simulink subsystem "Controller"  (R2025b)
settings: Solver=VariableStepAuto  StartTime=0.0  StopTime=10.0  RelTol=1e-3
values from neighbouring files (symbols this model uses):
  Feedforward = 0    [EReg_N2O_Simulink_Init.m]    (also in EReg_Tank_Drain_Init.m)
  K_D = 3    [EReg_N2O_Simulink_Init.m]    (also in EReg_Tank_Drain_Init.m = 8; EReg_Tank_Drain_N2O_Sim.m = params.K_D)
  K_I = 15    [EReg_N2O_Simulink_Init.m]    (also in EReg_Tank_Drain_Init.m = 2; EReg_Tank_Drain_N2O_Sim.m = params.K_I)
  K_P = 20    [EReg_N2O_Simulink_Init.m]    (also in EReg_Tank_Drain_Init.m = 8; EReg_Tank_Drain_N2O_Sim.m = params.K_P)
  N = 100    [EReg_N2O_Simulink_Init.m]    (also in EReg_Tank_Drain_Init.m)
libraries: simulink x2, slpidlib x1
settings Model: Creator=anzashoaib  LastModifiedBy=Rocklord

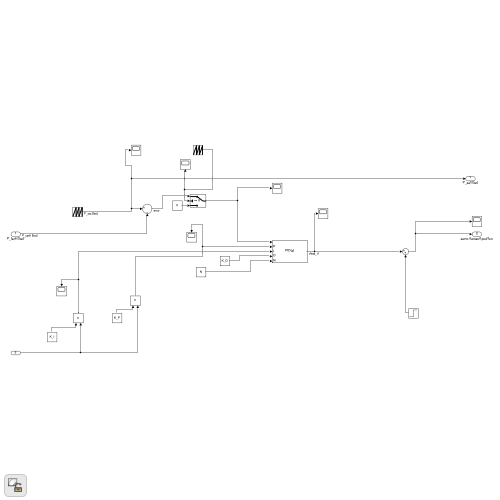
[thumbnail: Simulink's stored preview of the top-level diagram]
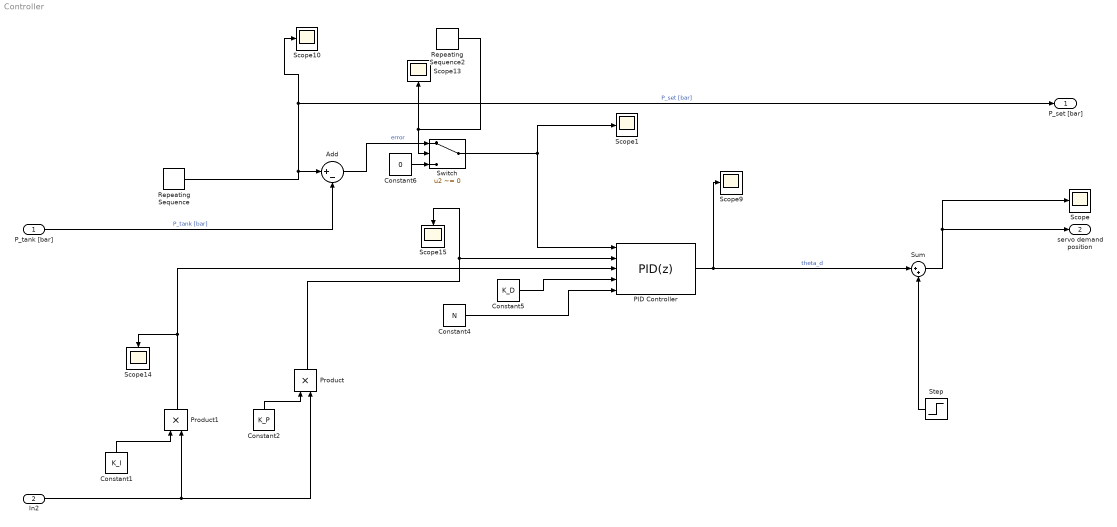
== system Controller ==
  P_tank [bar] : Inport  OutDataTypeStr=double  PortDimensions=1  SampleTime=0
  In2 : Inport  Port=2  OutDataTypeStr=double  PortDimensions=1  SampleTime=0
  Add : Sum  Inputs=|+-
  Constant1 : Constant  Value=K_I
  Constant2 : Constant  Value=K_P
  Constant4 : Constant  Value=N
  Constant5 : Constant  Value=K_D
  Constant6 : Constant  Value=0
  PID Controller : slpidlib/PID Controller  Controller=PID  Form=Parallel  TimeDomain=Discrete-time  UseExternalTs=off  SampleTime=-1  IntegratorMethod=Forward Euler  FilterMethod=Forward Euler  ControllerParametersSource=external  P=1.5  I=3  UseKiTs=off  D=0  UseExternalDerivativeSource=off  N=100  UseFilter=on  TunerSelectOption=Transfer Function Based (PID Tuner App)  InitialConditionSource=internal  InitialConditionForIntegrator=0  InitialConditionForFilter=0  DifferentiatorICPrevScaledInput=0  ExternalReset=none  TrackingMode=off  Kt=1  LimitOutput=off  SatLimitsSource=internal  UpperSaturationLimit=180  LowerSaturationLimit=0  LinearizeAsGain=on  AntiWindupMode=clamping  Kb=1  LimitIntegrator=on  UpperIntegratorSaturationLimit=20  LowerIntegratorSaturationLimit=-20  POutMin=[]  POutMax=[]  IOutMin=[]  IOutMax=[]  DOutMin=[]  DOutMax=[]  NOutMin=[]  NOutMax=[]  SumOutMin=[]  SumOutMax=[]  SaturationOutMin=[]  SaturationOutMax=[]  PParamMin=[]  PParamMax=[]  IParamMin=[]  IParamMax=[]  DParamMin=[]  DParamMax=[]  NParamMin=[]  NParamMax=[]  KbParamMin=[]  KbParamMax=[]  KtParamMin=[]  KtParamMax=[]  KbOutMin=[]  KbOutMax=[]  KtOutMin=[]  KtOutMax=[]  IntegratorOutMin=[]  IntegratorOutMax=[]  FilterOutMin=[]  FilterOutMax=[]  SumI1OutMin=[]  SumI1OutMax=[]  SumI2OutMin=[]  SumI2OutMax=[]  SumI3OutMin=[]  SumI3OutMax=[]  SumI4OutMin=[]  SumI4OutMax=[]  SumDOutMin=[]  SumDOutMax=[]  DifferentiatorOutMin=[]  DifferentiatorOutMax=[]  FilterDiffOutCoefMin=[]  FilterDiffOutCoefMax=[]  ReciprocalOutMin=[]  ReciprocalOutMax=[]  SumDenOutMin=[]  SumDenOutMax=[]  SumNumOutMin=[]  SumNumOutMax=[]  DivideOutMin=[]  DivideOutMax=[]  UdiffTsProdOutMin=[]  UdiffTsProdOutMax=[]  NTsProdOutMin=[]  NTsProdOutMax=[]  UintegralTsProdOutMin=[]  UintegralTsProdOutMax=[]  UngainTsProdOutMin=[]  UngainTsProdOutMax=[]  ClampingZeroOutDataTypeStr=Inherit: Inherit via back propagation  ClampingZeroOutMin=[]  ClampingZeroOutMax=[]  FilterDenConstantOutDataTypeStr=Inherit: Inherit via back propagation  FilterDenConstantOutMin=[]  FilterDenConstantOutMax=[]  PCopyOutDataTypeStr=Inherit: Inherit via back propagation  PCopyOutMin=[]  PCopyOutMax=[]  NCopyOutDataTypeStr=Inherit: Inherit via back propagation  NCopyOutMin=[]  NCopyOutMax=[]  IntegratorContinuousStateAttributes=''  IntegratorStateMustResolveToSignalObject=off  IntegratorRTWStateStorageClass=Auto  FilterContinuousStateAttributes=''  FilterStateMustResolveToSignalObject=off  FilterRTWStateStorageClass=Auto  ParallelPVariant=ExternalParameters  IdealPVariant=Disabled  IVariant=ExternalParameters  DVariant=ExternalParameters  IntegratorVariant=Discrete  SatVariant=Disabled  AWVariant=Passthrough  PCopyVariant=Disabled  TRVariant=Disabled  FdbkBlocksVariant=Forward  IdealPFdbkVariant=Disabled  SatFdbkVariant=Disabled  DerivativeFilterVariant=ForwardEulerFilter  NVariant=ExternalParameters  NCopyVariant=Disabled  FilterICVariant=InternalICsFilter  IntegratorICVariant=InternalICs  ExternalResetVariant=Disabled  TRSumVariant=Passthrough  SumFdbkVariant=Disabled  SumVariant=Sum_PID  TsampFilterVariant=InternalTs  TsampNgainVariant=Passthrough  TsampIntegralVariant=Disabled_SignalSpec  ExternalSaturationOutDataTypeStr=Inherit: Same as second input  DerivativeSourceVariant=ErrorSignal  PreIntVariant=InternalPreInt
  Product : Product
  Product1 : Product
  Repeating Sequence : simulink/Sources/Repeating Sequence  rep_seq_t=time  rep_seq_y=setpoint
  Repeating Sequence2 : simulink/Sources/Repeating Sequence  rep_seq_t=time  rep_seq_y=controller_on_setpoint
  Scope{,1,9..10,13..15} (7 alike) : Scope
      Scope settings: ActiveDisplayYMinimum=-1688.77171  ActiveDisplayYMaximum=357.47639  DataLoggingVariableName=ScopeData7
      Scope1 settings: ActiveDisplayYMinimum=-2.28363  ActiveDisplayYMaximum=0.62203  DataLoggingVariableName=ScopeData9
      Scope10 settings: ActiveDisplayYMinimum=51.3375  ActiveDisplayYMaximum=67.98472  DataLoggingVariableName=ScopeData10
      Scope13 settings: ActiveDisplayYMinimum=-0.125  ActiveDisplayYMaximum=1.125  DataLoggingVariableName=ScopeData11
      Scope14 settings: ActiveDisplayYMinimum=5.20102  ActiveDisplayYMaximum=13.19086  DataLoggingVariableName=ScopeData12
      Scope15 settings: ActiveDisplayYMinimum=13.00254  ActiveDisplayYMaximum=32.97714  DataLoggingVariableName=ScopeData13
      Scope9 settings: ActiveDisplayYMinimum=-1660.50954  ActiveDisplayYMaximum=362.9195  DataLoggingVariableName=ScopeData14
  Step : Step  After=Feedforward  SampleTime=0
  Sum : Sum  Inputs=|++
  Switch : Switch  Criteria=u2 ~= 0  SaturateOnIntegerOverflow=off  InputSameDT=off
  P_set [bar] : Outport  OutDataTypeStr=double  PortDimensions=1  SampleTime=0
  servo demand position : Outport  Port=2  OutDataTypeStr=double  PortDimensions=1  SampleTime=0
  wires:
  Product1/1 -> PID Controller/3, Scope14/1
  Product/1 -> PID Controller/2, Scope15/1
  Constant4/1 -> PID Controller/5
  Constant2/1 -> Product/1
  PID Controller/1 -> Sum/1, Scope9/1  "theta_d"
  P_tank [bar]/1 -> Add/2  "P_tank [bar]"
  Constant6/1 -> Switch/3
  Constant1/1 -> Product1/1
  In2/1 -> Product1/2, Product/2
  Step/1 -> Sum/2
  Constant5/1 -> PID Controller/4
  Repeating Sequence/1 -> Scope10/1, P_set [bar]/1, Add/1  "P_set [bar]"
  Add/1 -> Switch/1  "error"
  Switch/1 -> Scope1/1, PID Controller/1
  Repeating Sequence2/1 -> Scope13/1, Switch/2
  Sum/1 -> servo demand position/1, Scope/1
